simulink model "jacobs_test"  (R2022a)
settings: Solver=ode23s  StartTime=0.0  StopTime=10.0  FixedStep=0.01  RelTol=1e-3
values from neighbouring files (symbols this model uses):
  nx = 12 + 2*n    [nmpc_matlab.m]    (also in nmpc_test.m)
  ny = 8    [nmpc_matlab.m]    (also in nmpc_test.m)
  tau = [taub; taum]    [ee_dyn_check.m]
undefined symbols (not defined in the file or in its folder): fx, fy, fz, nz
settings Model: Creator=charl  LastModifiedBy=charl

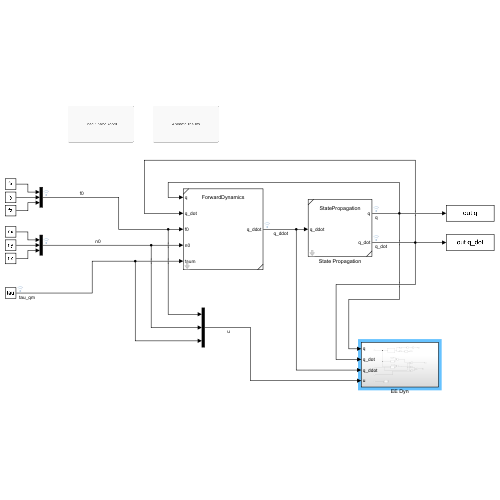
[thumbnail: Simulink's stored preview of the top-level diagram]
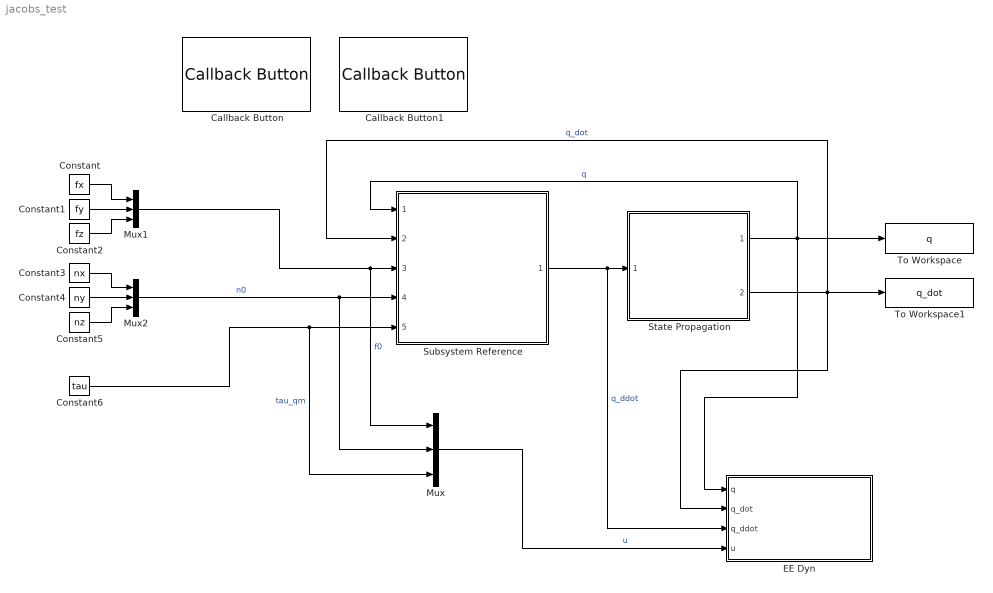
== system jacobs_test ==
  Callback Button : CallbackButton  ButtonText=Load SpaceRobot
      settings: ClickFcn=|
      | load('SC_2DoF.mat')
      | sc.homeConfig;
  Callback Button1 : CallbackButton  ButtonText=Animate results
      settings: ClickFcn=|
      | close all
      | sr.animate(out.q, 'fps', 17, 'rate', 1);
  Constant : Constant  Value=fx
  Constant1 : Constant  Value=fy
  Constant2 : Constant  Value=fz
  Constant3 : Constant  Value=nx
  Constant4 : Constant  Value=ny
  Constant5 : Constant  Value=nz
  Constant6 : Constant  Value=tau
  EE Dyn : Subsystem
  Mux : Mux  Inputs=3
  Mux1 : Mux  Inputs=3
  Mux2 : Mux  Inputs=3
  State Propagation : Subsystem  ReferencedSubsystem=StatePropagation  spaceRobot=sr  q_0=q_0  q_dot_0=q_dot_0
  Subsystem Reference : Subsystem  ReferencedSubsystem=ForwardDynamics  spaceRobot=sr  SimulateUsing=Interpreted execution
  To Workspace : ToWorkspace  VariableName=q  SaveFormat=Timeseries  SampleTime=-1
  To Workspace1 : ToWorkspace  VariableName=q_dot  SaveFormat=Timeseries  SampleTime=-1
  wires:
  Subsystem Reference/1 -> EE Dyn/3(q_ddot), State Propagation/1  "q_ddot"
  Mux2/1 -> Mux/2, Subsystem Reference/4  "n0"
  State Propagation/1 -> EE Dyn/1(q), Subsystem Reference/1, To Workspace/1  "q"
  State Propagation/2 -> EE Dyn/2(q_dot), To Workspace1/1, Subsystem Reference/2  "q_dot"
  Mux1/1 -> Mux/1, Subsystem Reference/3  "f0"
  Constant1/1 -> Mux1/2
  Constant2/1 -> Mux1/3
  Constant4/1 -> Mux2/2
  Constant5/1 -> Mux2/3
  Constant/1 -> Mux1/1
  Constant3/1 -> Mux2/1
  Constant6/1 -> Mux/3, Subsystem Reference/5  "tau_qm"
  Mux/1 -> EE Dyn/4(u)  "u"

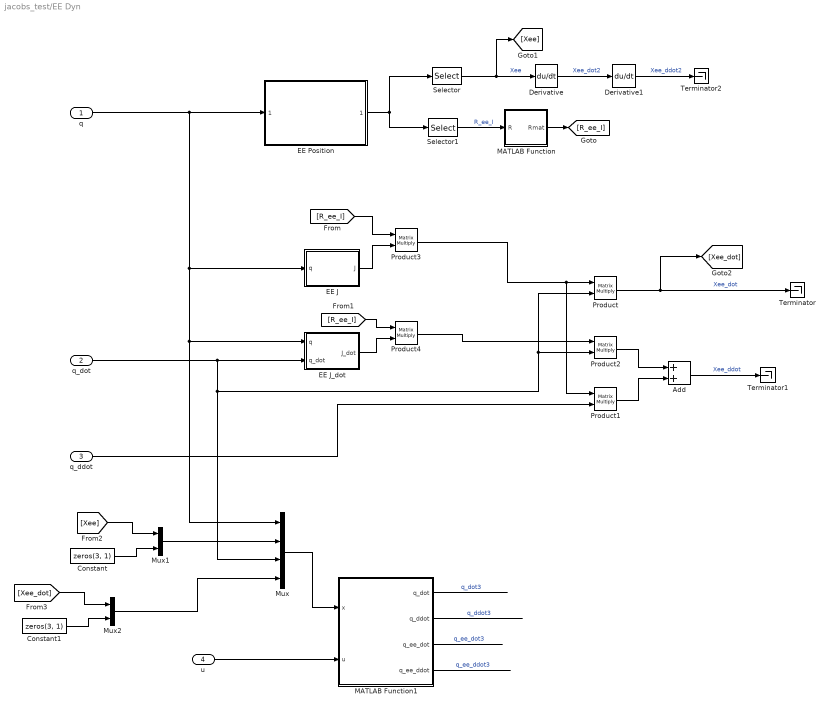
== system jacobs_test/EE Dyn ==
  q : Inport
  q_dot : Inport  Port=2
  q_ddot : Inport  Port=3
  u : Inport  Port=4
  Add : Sum
  Constant : Constant  Value=zeros(3, 1)
  Constant1 : Constant  Value=zeros(3, 1)
  Derivative : Derivative
  Derivative1 : Derivative
  EE J : MATLAB Function  TreatAsAtomicUnit=on
  EE J_dot : MATLAB Function  TreatAsAtomicUnit=on
  EE Position : Subsystem  ReferencedSubsystem=GetTransform  spaceRobot=sr  sourceBody=endeffector  targetBody=inertial  SimulateUsing=Interpreted execution
  MATLAB Function : MATLAB Function  TreatAsAtomicUnit=on
  MATLAB Function1 : MATLAB Function  TreatAsAtomicUnit=on
  Mux : Mux
  Mux1 : Mux  Inputs=2
  Mux2 : Mux  Inputs=2
  Product{,1..4} (5 alike) : Product  Multiplication=Matrix(*)
  Selector : Selector  NumberOfDimensions=2  InputPortWidth=[4 4]  IndexOptions=Index vector (dialog),Index vector (dialog)  Indices=[1:3],4  OutputSizes=1,1
  Selector1 : Selector  NumberOfDimensions=2  InputPortWidth=[4 4]  IndexOptions=Index vector (dialog),Index vector (dialog)  Indices=[1:3],[1:3]  OutputSizes=1,1
  Terminator : Terminator
  Terminator1 : Terminator
  Terminator2 : Terminator
  wires:
  Selector1/1 -> MATLAB Function/1(R)  "R_ee_I"
  Product3/1 -> Product1/1, Product/1
  q_dot/1 -> Mux/3, Product/2, Product2/2, EE J_dot/2(q_dot)
  EE J/1(J) -> Product3/2
  [R_ee_I] -> Product3/1
  Derivative1/1 -> Terminator2/1  "Xee_ddot2"
  Product2/1 -> Add/1
  Derivative/1 -> Derivative1/1  "Xee_dot2"
  EE Position/1 -> Selector1/1, Selector/1
  q/1 -> Mux/1, EE J_dot/1(q), EE J/1(q), EE Position/1
  Product1/1 -> Add/2
  Selector/1 -> [Xee], Derivative/1  "Xee"
  Product4/1 -> Product2/1
  MATLAB Function/1(Rmat) -> [R_ee_I]
  EE J_dot/1(J_dot) -> Product4/2
  Add/1 -> Terminator1/1  "Xee_ddot"
  Product/1 -> [Xee_dot], Terminator/1  "Xee_dot"
  [R_ee_I] -> Product4/1
  q_ddot/1 -> Product1/2
  u/1 -> MATLAB Function1/2(u)
  Mux1/1 -> Mux/2
  [Xee] -> Mux1/1
  Constant/1 -> Mux1/2
  [Xee_dot] -> Mux2/1
  Mux2/1 -> Mux/4
  Constant1/1 -> Mux2/2
  Mux/1 -> MATLAB Function1/1(x)
  MATLAB Function1/1(q_dot) -> ?  "q_dot3"
  MATLAB Function1/2(q_ddot) -> ?  "q_ddot3"
  MATLAB Function1/3(q_ee_dot) -> ?  "q_ee_dot3"
  MATLAB Function1/4(q_ee_ddot) -> ?  "q_ee_ddot3"

== matlab function jacobs_test/EE Dyn/EE J ==
  data: q input; J output
function J = fcn(q)
sr_info = SR2_info();

% 1 - Kinematics
[Rb, Ra, Rm] = RFunc_SR2(q);
Rm = reshape(Rm, 3, 3, []); % Split Rm to nk 3x3 arrays

% 2 - Kinetics
[~, ~, ~, A, ~] = Kin(sr_info, q, zeros(8, 1), zeros(8, 1), {Rb, Ra, Rm});

% 3 - J
J = Jacobian('endeffector', sr_info, A, {Rb, Ra});

% J_dot = Jacobian_dot('endeffector', sr_info, A, A_dot, {Rb, Ra}, wb, Omega);

end

== matlab function jacobs_test/EE Dyn/EE J_dot ==
  data: q input; J_dot output; q_dot input
function J_dot = fcn(q, q_dot)
sr_info = SR2_info();

% 1 - Kinematics
[Rb, Ra, Rm] = RFunc_SR2(q);
Rm = reshape(Rm, 3, 3, []); % Split Rm to nk 3x3 arrays

% 2 - Kinetics
[t, ~, Omega, A, A_dot] = Kin(sr_info, q, q_dot, zeros(8, 1), {Rb, Ra, Rm});
wb = t{1}(4:6);

% 3 - J_dot
J_dot = Jacobian_dot('endeffector', sr_info, A, A_dot, {Rb, Ra}, wb, Omega);

== matlab function jacobs_test/EE Dyn/MATLAB Function ==
  data: R input; Rmat output
function Rmat = fcn(R)

Rmat = blkdiag(R, R);

== matlab function jacobs_test/EE Dyn/MATLAB Function1 ==
  data: x input; u input; q_dot output; q_ddot output; q_ee_dot output; q_ee_ddot output
function [q_dot, q_ddot, q_ee_dot, q_ee_ddot] = fcn(x, u)

dx = sr_ee_state_func(x, u);

q_dot = dx(1:8);
q_ee_dot = dx(9:14) ;

q_ddot = dx(15:22);
q_ee_ddot = dx(23:28);
